simulink model "induction_machine_harness"  (R2016a)
settings: Solver=ode45  StartTime=start_time  StopTime=stop_time  MaxStep=max_step_size  RelTol=1e-3
values from neighbouring files (symbols this model uses):
  D = 0    [induction_machine_script.m]
  H = 0.5    [induction_machine_script.m]
  K1 = 0    [induction_machine_script.m]    (also in induction_machine_ssop.m = varargin{1}; end)
  K2 = 0    [induction_machine_script.m]    (also in induction_machine_ssop.m = varargin{2}; end)
  P = 6    [induction_machine_script.m]
  phvs = 0    [induction_machine_script.m]
  Tbase = Prated/(2/P*wbase)    [induction_machine_per_unit_bases.m]
  th0_pu = 0    [induction_machine_script.m]
  the0_pu = 0    [induction_machine_script.m]
  thr0_pu = 0    [induction_machine_script.m]
  wbase = 2*pi*frated    [induction_machine_per_unit_bases.m]
  wr0_pu = 0    [induction_machine_script.m]
settings Model: Creator=Jeff Mayer  LastModifiedBy=Seth Barger
settings DataIOCC: LimitDataPoints=on  SaveFormat=Array  SignalLoggingSaveFormat=ModelDataLogs
settings OptimizationCC: DefaultParameterBehavior=Inlined  ExpressionDepthLimit=2147483647
settings DebuggingCC: UnderspecifiedInitializationDetection=Classic  MergeDetectMultiDrivingBlocksExec=none  SolverPrmCheckMsg=warning  FcnCallInpInsideContextMsg=UseLocalSettings  StateNameClashWarn=warning
settings HardwareCC: ProdBitPerPointer=32  ProdLargestAtomicFloat=None  ProdIntDivRoundTo=Undefined  ProdEndianess=Unspecified  ProdWordSize=32  ProdHWDeviceType=32-bit Generic
settings ModelReferenceCC: ModelReferenceNumInstancesAllowed=Single  PropagateSignalLabelsOutOfModel=off
settings SFSimCC: SimParseCustomCode=off
settings GRTTargetCC: CombineOutputUpdateFcns=off  GRTInterface=on
settings ConfigComp: CovModelRefEnable=Off

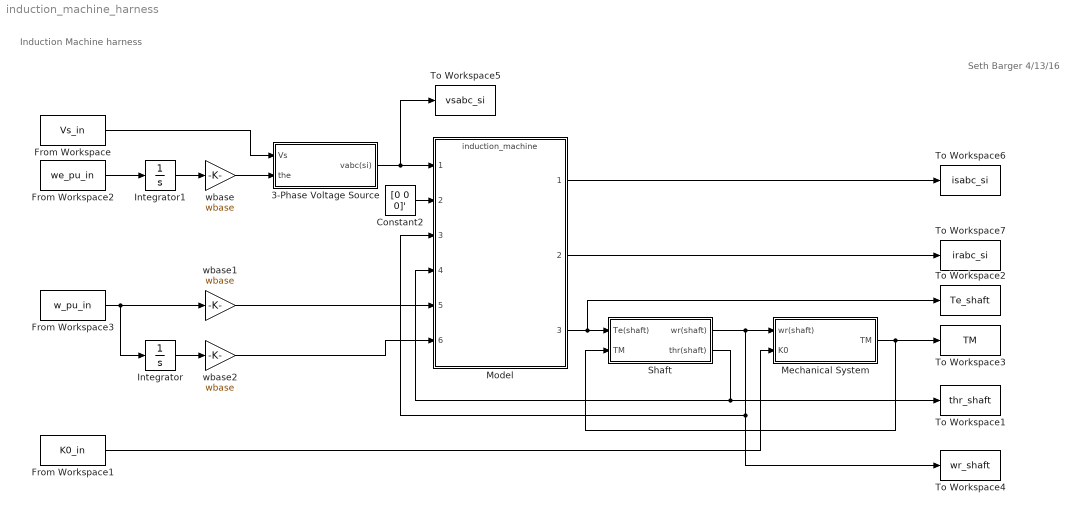
== system induction_machine_harness ==
  note: Seth Barger
      | 4/13/16
  note: Induction Machine harness
  3-Phase Voltage Source : Subsystem
  Constant2 : Constant  Value=[0 0 0]'
  From Workspace : FromWorkspace  VariableName=Vs_in  SampleTime=0  Interpolate=off  OutputAfterFinalValue=Holding final value
  From Workspace1 : FromWorkspace  VariableName=K0_in  SampleTime=0  Interpolate=off  OutputAfterFinalValue=Holding final value
  From Workspace2 : FromWorkspace  VariableName=we_pu_in  SampleTime=0  Interpolate=off  OutputAfterFinalValue=Holding final value
  From Workspace3 : FromWorkspace  VariableName=w_pu_in  SampleTime=0  Interpolate=off  OutputAfterFinalValue=Holding final value
  Integrator : Integrator  InitialCondition=th0_pu
  Integrator1 : Integrator  InitialCondition=the0_pu
  Mechanical System : Subsystem
  Model : ModelReference  ModelNameDialog=induction_machine  SimulationMode=Normal  ModelReferenceVersion=1.7
  Shaft : Subsystem
  To Workspace1 : ToWorkspace  VariableName=thr_shaft  SampleTime=-1
  To Workspace2 : ToWorkspace  VariableName=Te_shaft  SampleTime=-1
  To Workspace3 : ToWorkspace  VariableName=TM  SampleTime=-1
  To Workspace4 : ToWorkspace  VariableName=wr_shaft  SampleTime=-1
  To Workspace5 : ToWorkspace  VariableName=vsabc_si  SampleTime=-1
  To Workspace6 : ToWorkspace  VariableName=isabc_si  SampleTime=-1
  To Workspace7 : ToWorkspace  VariableName=irabc_si  SampleTime=-1
  wbase : Gain  Gain=wbase
  wbase1 : Gain  Gain=wbase
  wbase2 : Gain  Gain=wbase
  wires:
  Shaft/1(wr(shaft)) -> Mechanical System/1(wr(shaft)), Model/3, To Workspace4/1
  Shaft/2(thr(shaft)) -> Model/4, To Workspace1/1
  Constant2/1 -> Model/2
  Integrator/1 -> wbase2/1
  From Workspace2/1 -> Integrator1/1
  3-Phase Voltage Source/1(vabc(si)) -> Model/1, To Workspace5/1
  Integrator1/1 -> wbase/1
  wbase1/1 -> Model/5
  wbase2/1 -> Model/6
  Mechanical System/1(TM) -> Shaft/2(TM), To Workspace3/1
  wbase/1 -> 3-Phase Voltage Source/2(the)
  From Workspace1/1 -> Mechanical System/2(K0)
  From Workspace3/1 -> wbase1/1, Integrator/1
  From Workspace/1 -> 3-Phase Voltage Source/1(Vs)
  Model/1 -> To Workspace6/1
  Model/2 -> To Workspace7/1
  Model/3 -> To Workspace2/1, Shaft/1(Te(shaft))

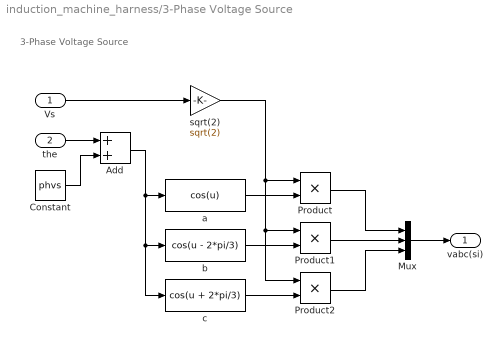
== system induction_machine_harness/3-Phase Voltage Source ==
  note: 3-Phase Voltage Source
  Vs : Inport
  the : Inport  Port=2
  Add : Sum
  Constant : Constant  Value=phvs
  Mux : Mux  Inputs=3
  Product : Product  RndMeth=Zero
  Product1 : Product  RndMeth=Zero
  Product2 : Product  RndMeth=Zero
  a : Fcn  Expr=cos(u)
  b : Fcn  Expr=cos(u - 2*pi/3)
  c : Fcn  Expr=cos(u + 2*pi/3)
  sqrt(2) : Gain  Gain=sqrt(2)
  vabc(si) : Outport
  wires:
  sqrt(2)/1 -> Product2/1, Product1/1, Product/1
  a/1 -> Product/2
  b/1 -> Product1/2
  c/1 -> Product2/2
  Product/1 -> Mux/1
  Product1/1 -> Mux/2
  Product2/1 -> Mux/3
  Mux/1 -> vabc(si)/1
  Add/1 -> a/1, b/1, c/1
  the/1 -> Add/1
  Constant/1 -> Add/2
  Vs/1 -> sqrt(2)/1

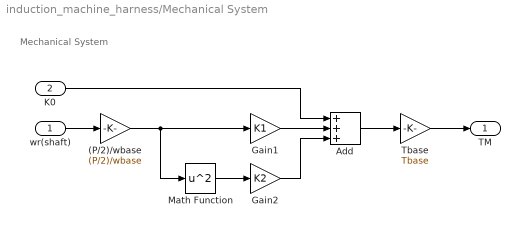
== system induction_machine_harness/Mechanical System ==
  note: Mechanical System
  wr(shaft) : Inport
  K0 : Inport  Port=2
  (P/2)/wbase : Gain  Gain=(P/2)/wbase
  Add : Sum  Inputs=+++
  Gain1 : Gain  Gain=K1
  Gain2 : Gain  Gain=K2
  Math Function : Math  Operator=square  SaturateOnIntegerOverflow=on
  Tbase : Gain  Gain=Tbase
  TM : Outport
  wires:
  Gain1/1 -> Add/2
  K0/1 -> Add/1
  Gain2/1 -> Add/3
  Math Function/1 -> Gain2/1
  Add/1 -> Tbase/1
  Tbase/1 -> TM/1
  (P/2)/wbase/1 -> Gain1/1, Math Function/1
  wr(shaft)/1 -> (P/2)/wbase/1

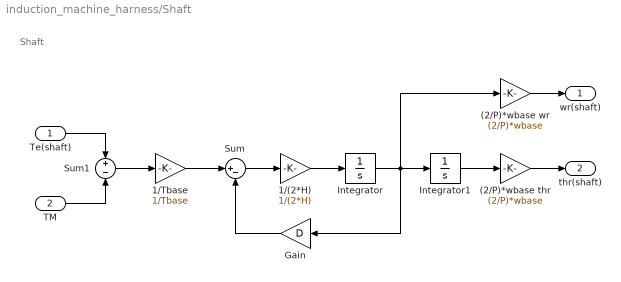
== system induction_machine_harness/Shaft ==
  note: Shaft
  Te(shaft) : Inport
  TM : Inport  Port=2
  (2/P)*wbase thr : Gain  Gain=(2/P)*wbase
  (2/P)*wbase wr : Gain  Gain=(2/P)*wbase
  1/(2*H) : Gain  Gain=1/(2*H)
  1/Tbase : Gain  Gain=1/Tbase
  Gain : Gain  Gain=D
  Integrator : Integrator  InitialCondition=wr0_pu
  Integrator1 : Integrator  InitialCondition=thr0_pu
  Sum : Sum  Inputs=|+-
  Sum1 : Sum  Inputs=+|-
  wr(shaft) : Outport
  thr(shaft) : Outport  Port=2
  wires:
  Sum/1 -> 1/(2*H)/1
  1/(2*H)/1 -> Integrator/1
  Integrator/1 -> Gain/1, (2/P)*wbase wr/1, Integrator1/1
  Integrator1/1 -> (2/P)*wbase thr/1
  Te(shaft)/1 -> Sum1/1
  (2/P)*wbase wr/1 -> wr(shaft)/1
  (2/P)*wbase thr/1 -> thr(shaft)/1
  Gain/1 -> Sum/2
  TM/1 -> Sum1/2
  Sum1/1 -> 1/Tbase/1
  1/Tbase/1 -> Sum/1
